simulink model "GlobalMPC"  (R2022b)
settings: Solver=FixedStepAuto  StartTime=0.0  FixedStep=3600  RelTol=1e-3
values from neighbouring files (symbols this model uses):
  c = scaled_standard_constants    [Run_simulation.m]
settings Model: Creator=is123  LastModifiedBy=is123
settings OptimizationCC: ReuseModelBlockBuffer=on

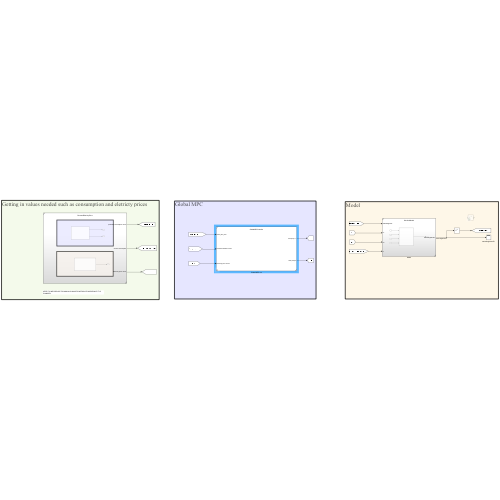
[thumbnail: Simulink's stored preview of the top-level diagram]
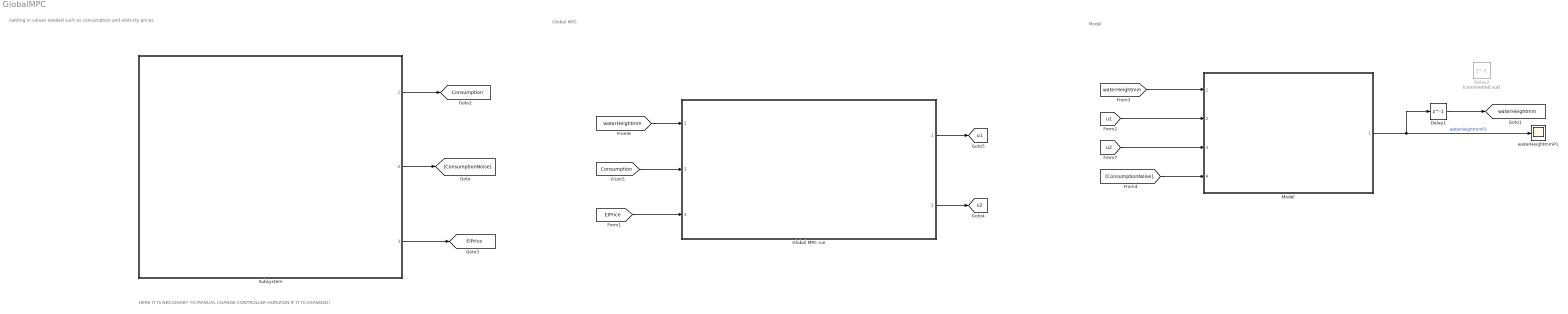
== system GlobalMPC ==
  note: Getting in values needed such as consumption and eletricty prices
  note: Global MPC
  note: Model
  note: HERE IT IS NECCESARY TO MANUAL CHANGE CONTROLLER HORIZION IF IT IS CHANGED!
  Delay1 : Delay  DelayLength=1  InitialCondition=c.V/c.At*1e3
  Delay2 : Delay  Commented=on  DelayLength=1  InitialCondition=534
  Global MPC run : Subsystem  ReferencedSubsystem=GlobalMPController  c=scaled_standard_constants
  Model : Subsystem  ReferencedSubsystem=SimulinkModel
  Subsystem : Subsystem  ReferencedSubsystem=DemandEletricityPrice
  waterHeightmmP1 : Scope
  tag scope: Consumption=global, ElPrice=global, u1=global, u2=global, waterHeightmm=global
  wires:
  Model/1 -> Delay1/1, waterHeightmmP1/1  "waterHeightmmP1"
  [waterHeightmm] -> Model/1
  [u1] -> Model/2
  [ConsumptionNoise] -> Model/4
  Global MPC run/1 -> [u1]
  Subsystem/2 -> [ConsumptionNoise]
  Subsystem/1 -> [Consumption]
  Subsystem/3 -> [ElPrice]
  [waterHeightmm] -> Global MPC run/1
  [Consumption] -> Global MPC run/2
  [ElPrice] -> Global MPC run/3
  Global MPC run/2 -> [u2]
  [u2] -> Model/3
  Delay1/1 -> [waterHeightmm]
